simulink subsystem "apply_actual_conditions"  (R2020a)
settings: Solver=VariableStepAuto  StartTime=0.0  StopTime=10.0  RelTol=1e-3
settings Model: Creator=upattacini  LastModifiedBy=upattacini

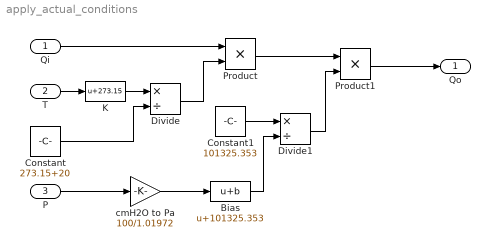
== system apply_actual_conditions ==
  Qi : Inport
  T : Inport  Port=2
  P : Inport  Port=3
  Bias : Bias  Bias=101325.353
  Constant : Constant  Value=273.15+20  OutDataTypeStr=single
  Constant1 : Constant  Value=101325.353  OutDataTypeStr=single
  Divide : Product  Inputs=*/
  Divide1 : Product  Inputs=*/
  K : Bias  Bias=273.15
  Product : Product
  Product1 : Product
  cmH2O to Pa : Gain  Gain=100/1.01972
  Qo : Outport
  wires:
  Qi/1 -> Product/1
  Product/1 -> Product1/1
  Product1/1 -> Qo/1
  Divide/1 -> Product/2
  Divide1/1 -> Product1/2
  Constant1/1 -> Divide1/1
  cmH2O to Pa/1 -> Bias/1
  P/1 -> cmH2O to Pa/1
  T/1 -> K/1
  Constant/1 -> Divide/2
  K/1 -> Divide/1
  Bias/1 -> Divide1/2
